simulink model "MG2Controller_Observer1"  (R2021a)
settings: Solver=VariableStepAuto  StartTime=0.0  StopTime=400  RelTol=1e-3
settings Model: Creator=isaacito  LastModifiedBy=isaacito

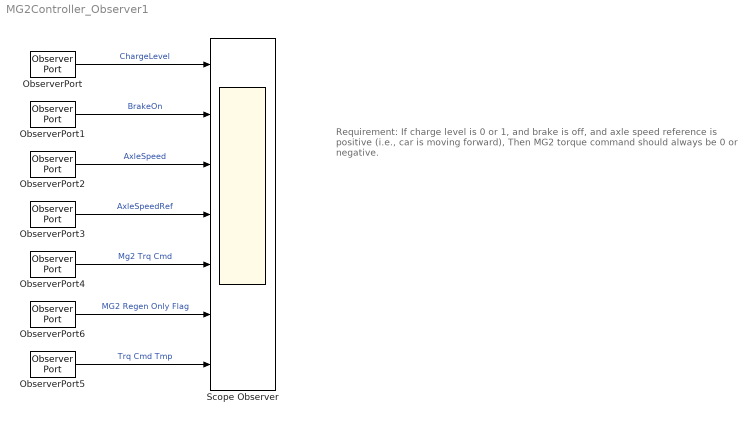
== system MG2Controller_Observer1 ==
  note: Requirement:
      |
      | If
      | charge level is 0 or 1,
      | and
      | brake is off,
      | and
      | axle speed reference is positive (i.e., car is moving forward),
      |
      | Then
      | MG2 torque command should always be 0 or negative.
  ObserverPort{,1..6} (7 alike) : ObserverPort
  Scope Observer : Scope  NumInputPorts=7
  wires:
  ObserverPort/1 -> Scope Observer/1  "ChargeLevel"
  ObserverPort1/1 -> Scope Observer/2  "BrakeOn"
  ObserverPort2/1 -> Scope Observer/3  "AxleSpeed"
  ObserverPort3/1 -> Scope Observer/4  "AxleSpeedRef"
  ObserverPort4/1 -> Scope Observer/5  "Mg2 Trq Cmd"
  ObserverPort6/1 -> Scope Observer/6  "MG2 Regen Only Flag"
  ObserverPort5/1 -> Scope Observer/7  "Trq Cmd Tmp"
